simulink model "MAS_All"  (R2021b)
settings: Solver=ode23t  StartTime=0.0  StopTime=100  MaxStep=1e-2  MinStep=1e-6  RelTol=1e-3
StopFcn:
  | %plotUnicycles(L,out)
undefined symbols (not defined in the file): b, deltaNoise, fieldParams, fminmax, fRef, grad_sel, IC, Kd, KLFR, Kp, Lap, m
settings Model: SimulationMode=accelerator  Creator=JanaTonio  LastModifiedBy=JanaTonio

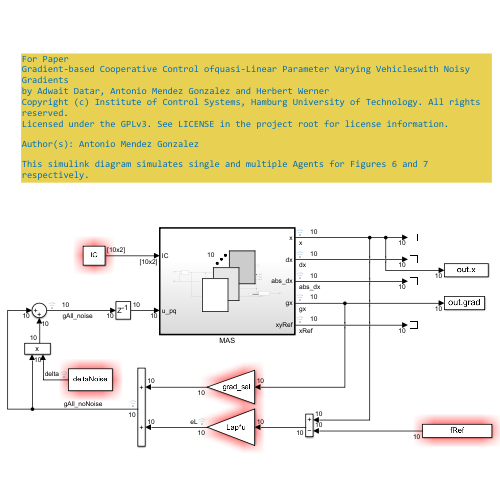
[thumbnail: Simulink's stored preview of the top-level diagram]
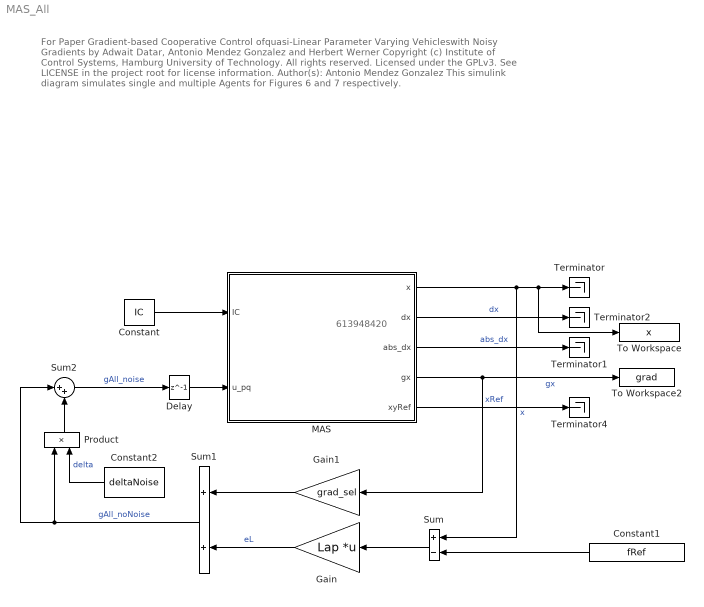
== system MAS_All ==
  note: For Paper
      | Gradient-based Cooperative Control ofquasi-Linear Parameter Varying Vehicleswith Noisy Gradients
      | by Adwait Datar, Antonio Mendez Gonzalez and Herbert Werner
      | Copyright (c) Institute of Control Systems, Hamburg University of Technology. All rights reserved.
      | Licensed under the GPLv3. See LICENSE in the project root for license information.
      |
      | Author(s): Antonio Mendez Gonzalez
      |
      | This simulink diagram simulates single and multiple Agents for Figures 6 and 7 respectively.
  note: 613948420
  Constant : Constant  Value=IC  VectorParams1D=off
  Constant1 : Constant  Value=fRef
  Constant2 : Constant  Value=deltaNoise
  Delay : Delay  DelayLength=1
  Gain : Gain  Gain=Lap  Multiplication=Matrix(K*u)
  Gain1 : Gain  Gain=grad_sel
  MAS : Subsystem  TreatAsAtomicUnit=on
  Product : Product
  Sum : Sum  Inputs=+-
  Sum1 : Sum
  Sum2 : Sum  Inputs=|++
  Terminator{,1..2,4} (4 alike) : Terminator
  To Workspace : ToWorkspace  VariableName=x  SampleTime=-1
      settings: Save2DSignal=2-D array (concatenate along first dimension)
  To Workspace2 : ToWorkspace  VariableName=grad  SampleTime=-1
      settings: Save2DSignal=2-D array (concatenate along first dimension)
  wires:
  MAS/2(dx) -> Terminator2/1  "dx"
  MAS/1(x) -> To Workspace/1, Terminator/1, Sum/1  "x"
  MAS/3(abs_dx) -> Terminator1/1  "abs_dx"
  Constant/1 -> MAS/1(IC)
  Sum/1 -> Gain/1
  Delay/1 -> MAS/2(u_pq)
  MAS/5(xyRef) -> Terminator4/1  "xRef"
  Gain/1 -> Sum1/2  "eL"
  MAS/4(gx) -> Gain1/1, To Workspace2/1  "gx"
  Sum1/1 -> Sum2/1, Product/1  "gAll_noNoise"
  Sum2/1 -> Delay/1  "gAll_noise"
  Gain1/1 -> Sum1/1
  Constant1/1 -> Sum/2
  Constant2/1 -> Product/2  "delta"
  Product/1 -> Sum2/2

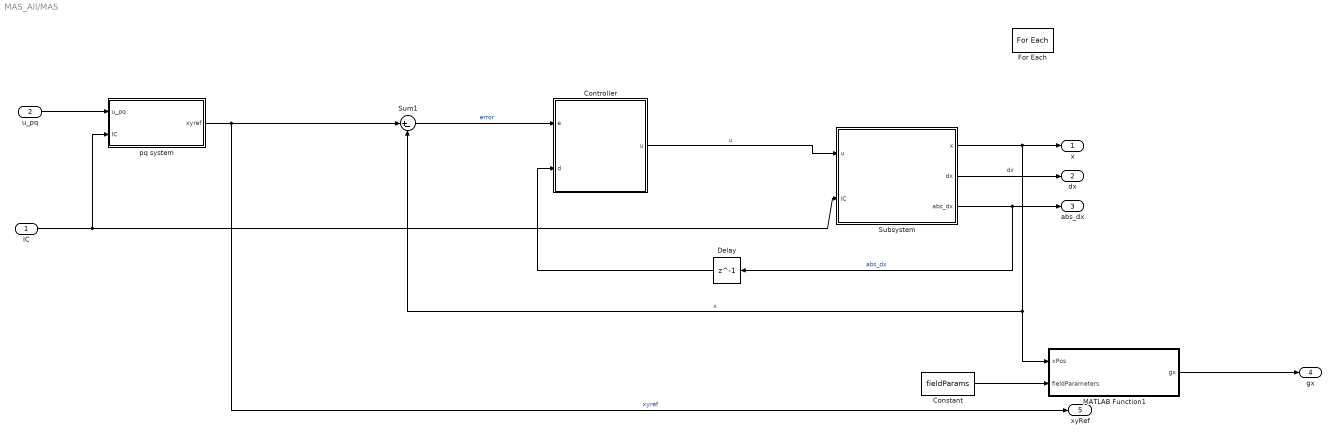
== system MAS_All/MAS ==
  IC : Inport  Partition=on  PartitionDimension=1  PartitionWidth=1  PartitionOffset=0
  u_pq : Inport  Port=2  Partition=on  PartitionDimension=1  PartitionWidth=1  PartitionOffset=0
  Constant : Constant  Value=fieldParams  OutDataTypeStr=Bus: fieldParamsBus
  Controller : Subsystem  mask{P=KLFR}
      mask prompts: P "Controller Structure"
  Delay : Delay  DelayLength=1
  For Each : ForEach  DisableCoverage=on
  MATLAB Function1 : MATLAB Function  TreatAsAtomicUnit=on
  Subsystem : Subsystem
  Sum1 : Sum  Inputs=|+-
  pq system : Subsystem
  x : Outport  PortDimensions=1  ConcatenationDimension=1
  dx : Outport  Port=2  PortDimensions=1  ConcatenationDimension=1
  abs_dx : Outport  Port=3  PortDimensions=1  ConcatenationDimension=1
  gx : Outport  Port=4  PortDimensions=1  ConcatenationDimension=1
  xyRef : Outport  Port=5  PortDimensions=1  ConcatenationDimension=1
  wires:
  u_pq/1 -> pq system/1(u_pq)
  pq system/1(xyref) -> xyRef/1, Sum1/1  "xyref"
  Subsystem/1(x) -> MATLAB Function1/1(xPos), Sum1/2, x/1  "x"
  Delay/1 -> Controller/2(d)
  Controller/1(u) -> Subsystem/1(u)  "u"
  IC/1 -> pq system/2(IC), Subsystem/2(IC)
  Subsystem/2(dx) -> dx/1  "dx"
  Sum1/1 -> Controller/1(e)  "error"
  Constant/1 -> MATLAB Function1/2(fieldParameters)
  MATLAB Function1/1(gx) -> gx/1
  Subsystem/3(abs_dx) -> Delay/1, abs_dx/1  "abs_dx"

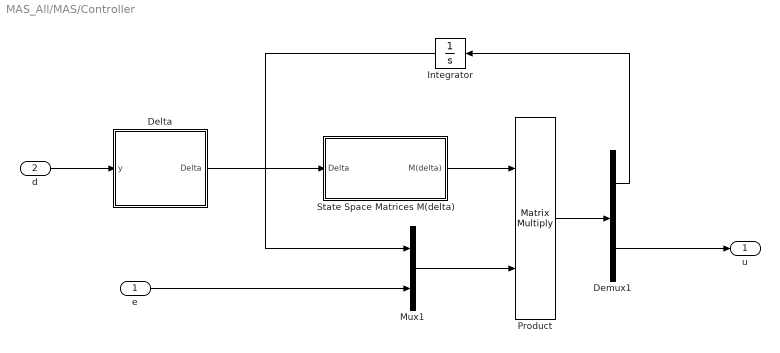
== system MAS_All/MAS/Controller ==
  e : Inport
  d : Inport  Port=2
  Delta : Subsystem
      mask Display:
      | patch([0.2 .5 0.8], [0.2 0.8 0.2], [0 0 0])
      | patch([0.25 .5 0.75], [0.25 0.75 0.25], [1 1 1])
  Demux1 : Demux  Outputs=[size(P.A, 1); size(P.C_y, 1)]
  Integrator : Integrator
  Mux1 : Mux  Inputs=2
  Product : Product  Multiplication=Matrix(*)  RndMeth=Zero
  State Space Matrices M(delta) : Subsystem
  u : Outport
  wires:
  State Space Matrices M(delta)/1(M(delta)) -> Product/1
  d/1 -> Delta/1(y)
  Demux1/2 -> u/1
  Integrator/1 -> Mux1/1
  Mux1/1 -> Product/2
  Demux1/1 -> Integrator/1
  Delta/1(Delta) -> State Space Matrices M(delta)/1(Delta)
  e/1 -> Mux1/2
  Product/1 -> Demux1/1

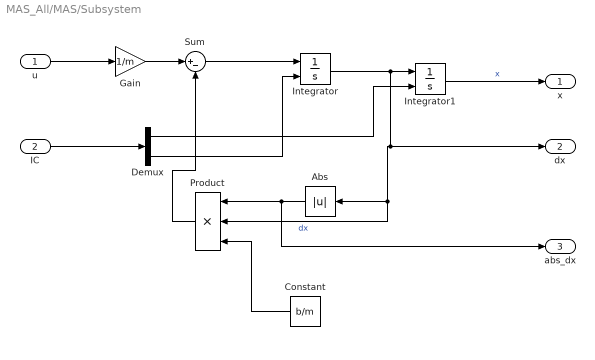
== system MAS_All/MAS/Subsystem ==
  u : Inport
  IC : Inport  Port=2
  Abs : Abs
  Constant : Constant  Value=b/m
  Demux : Demux  Outputs=2
  Gain : Gain  Gain=1/m
  Integrator : Integrator  InitialConditionSource=external
  Integrator1 : Integrator  InitialConditionSource=external
  Product : Product  Inputs=3
  Sum : Sum  Inputs=|+-
  x : Outport
  dx : Outport  Port=2
  abs_dx : Outport  Port=3
  wires:
  u/1 -> Gain/1
  IC/1 -> Demux/1
  Integrator1/1 -> x/1  "x"
  Integrator/1 -> Product/2, Abs/1, dx/1, Integrator1/1  "dx"
  Abs/1 -> abs_dx/1, Product/1
  Gain/1 -> Sum/1
  Demux/1 -> Integrator1/2
  Demux/2 -> Integrator/2
  Sum/1 -> Integrator/1
  Constant/1 -> Product/3
  Product/1 -> Sum/2

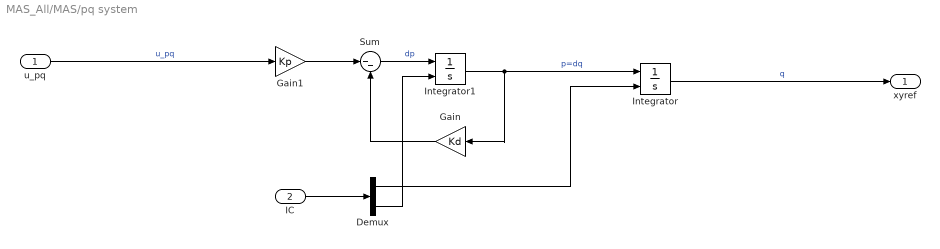
== system MAS_All/MAS/pq system ==
  u_pq : Inport
  IC : Inport  Port=2
  Demux : Demux  Outputs=2
  Gain : Gain  Gain=Kd
  Gain1 : Gain  Gain=Kp
  Integrator : Integrator  InitialConditionSource=external  InitialCondition=IC(1,1)
  Integrator1 : Integrator  InitialConditionSource=external
  Sum : Sum  Inputs=|--
  xyref : Outport
  wires:
  Integrator1/1 -> Integrator/1, Gain/1  "p=dq"
  Sum/1 -> Integrator1/1  "dp"
  Gain1/1 -> Sum/1
  Gain/1 -> Sum/2
  Integrator/1 -> xyref/1  "q"
  u_pq/1 -> Gain1/1  "u_pq"
  IC/1 -> Demux/1
  Demux/1 -> Integrator/2
  Demux/2 -> Integrator1/2

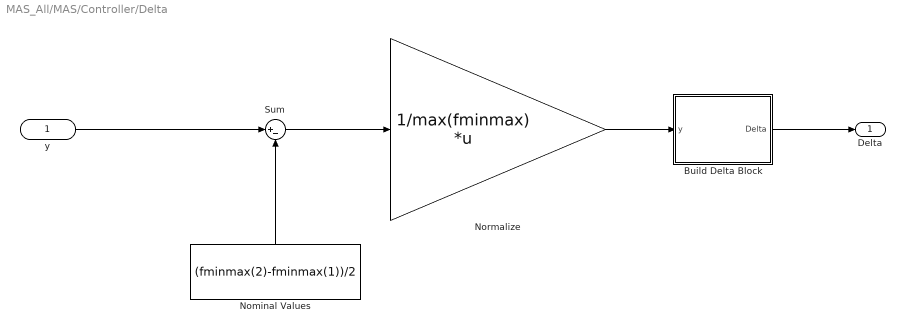
== system MAS_All/MAS/Controller/Delta ==
  y : Inport
  Build Delta Block : MATLAB Function  TreatAsAtomicUnit=on
  Nominal Values : Constant  Value=(fminmax(2)-fminmax(1))/2  VectorParams1D=off
  Normalize : Gain  Gain=1/max(fminmax)  Multiplication=Matrix(K*u) (u vector)
  Sum : Sum  Inputs=|+-
  Delta : Outport
  wires:
  Build Delta Block/1(Delta) -> Delta/1
  Sum/1 -> Normalize/1
  Nominal Values/1 -> Sum/2
  Normalize/1 -> Build Delta Block/1(y)
  y/1 -> Sum/1

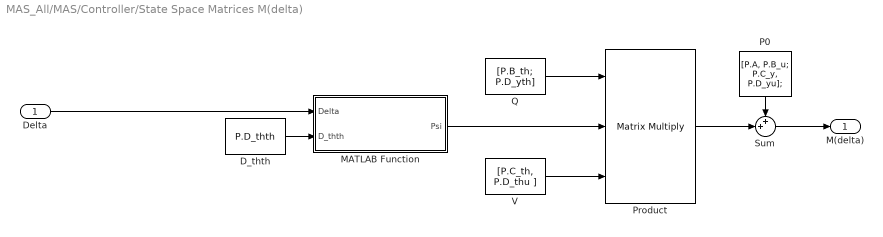
== system MAS_All/MAS/Controller/State Space Matrices M(delta) ==
  Delta : Inport
  D_thth : Constant  Value=P.D_thth
  MATLAB Function : MATLAB Function  TreatAsAtomicUnit=on
  P0 : Constant  Value=[P.A, P.B_u; P.C_y, P.D_yu];  VectorParams1D=off
  Product : Product  Inputs=3  Multiplication=Matrix(*)  RndMeth=Zero
  Q : Constant  Value=[P.B_th; P.D_yth]
  Sum : Sum  Inputs=++|
  V : Constant  Value=[P.C_th, P.D_thu ]  VectorParams1D=off
  M(delta) : Outport
  wires:
  MATLAB Function/1(Psi) -> Product/2
  Delta/1 -> MATLAB Function/1(Delta)
  V/1 -> Product/3
  Sum/1 -> M(delta)/1
  P0/1 -> Sum/1
  Product/1 -> Sum/2
  Q/1 -> Product/1
  D_thth/1 -> MATLAB Function/2(D_thth)

== matlab function MAS_All/MAS/MATLAB Function1 ==
  data: xPos input; gx output; fieldParameters input
function gx = gradPsi(xPos, fieldParameters)

xM = fieldParameters.xM;

L_psi = fieldParameters.L_psi;

gx = -L_psi*(xM - xPos);

end

== matlab function MAS_All/MAS/Controller/Delta/Build Delta Block ==
  data: y input; Delta output
function Delta = Delta(y)
%#codegen

Delta = diag([y(1)]);

== matlab function MAS_All/MAS/Controller/State Space Matrices M(delta)/MATLAB Function ==
  data: Delta input; Psi output; D_thth input
function Psi = Psi(Delta, D_thth)
%#codegen

[nwth, nzth] = size(Delta);

Psi = Delta * (eye(nwth) - D_thth*Delta)^-1;
